simulink model "Simulation"  (R2014a)
settings: Solver=ode3  SolverMode=SingleTasking  StartTime=0.0  StopTime=5000.0  RelTol=1e-3
settings Model: ExtModeTrigDuration=2  Creator=beaverl  LastModifiedBy=beaverl
settings OptimizationCC: OptimizeModelRefInitCode=on  LifeSpan=1
settings DebuggingCC: UnderspecifiedInitializationDetection=Classic  SolverPrmCheckMsg=none
settings HardwareCC: ProdBitPerInt=16  ProdBitPerPointer=8  ProdIntDivRoundTo=Zero  ProdEndianess=LittleEndian  ProdWordSize=8  ProdHWDeviceType=Atmel->AVR
settings RTWCC: SystemTargetFile=realtime.tlc  GenerateMakefile=off  TemplateMakefile=realtime.tmf  Description=Run on Target Hardware  RTWVerbose=off  ProcessScript=realtime_make_rtw_hook
settings STFCustomTargetCC: TargetLibSuffix=.a  GenerateSampleERTMain=on  ConcurrentExecutionCompliant=off  GeneratePreprocessorConditionals=Use local settings  ERTCustomFileBanners=on  SupportNonInlinedSFcns=off  SupportVariableSizeSignals=on  MATLABClassNameForMDSCustomization=Simulink.SoftwareTarget.ERTCustomization  GRTInterface=off  SystemTargetFile=realtime.tlc
settings ERTTargetCC: CombineOutputUpdateFcns=off  SupportContinuousTime=on  SupportVariableSizeSignals=on  ExtModeTransport=3  ExtModeMexFile=ext_serial_win32_comm  ExtModeMexArgs=0 1 9600  ERTSrcFileBannerTemplate=realtime_code_template.cgt  ERTHdrFileBannerTemplate=realtime_code_template.cgt  ERTDataSrcFileTemplate=realtime_code_template.cgt  ERTDataHdrFileTemplate=realtime_code_template.cgt  ERTCustomFileTemplate=realtime_file_process.tlc

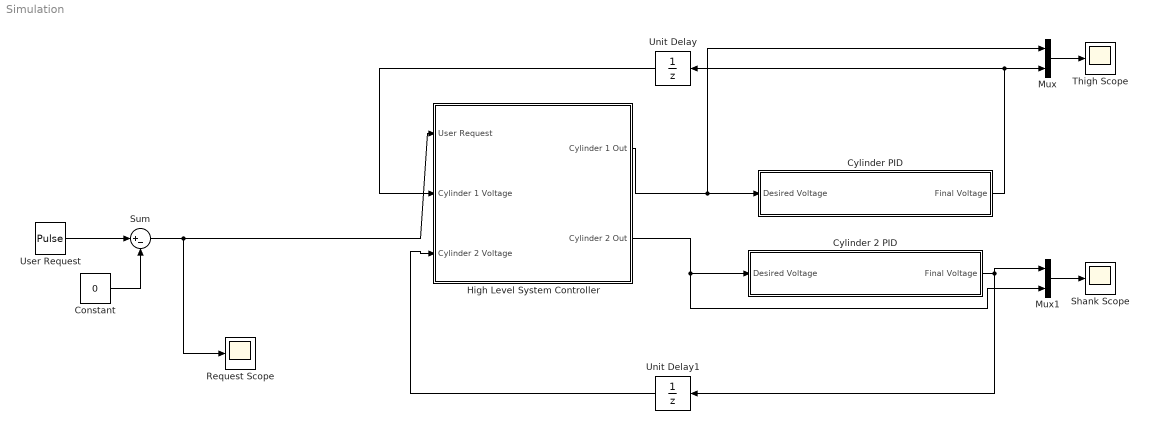
== system Simulation ==
  Constant : Constant  Value=0
  Cylinder 2 PID : Subsystem
  Cylinder PID : Subsystem
  High Level System Controller : Subsystem
  Mux : Mux  Inputs=2
  Mux1 : Mux  Inputs=2
  Request Scope : Scope
      settings: TimeRange=1  YMin=0.95  YMax=1.05
  Shank Scope : Scope
      settings: TimeRange=1  YMin=1.88  YMax=2  SaveName=ScopeData6
  Sum : Sum  Inputs=|+-
  Thigh Scope : Scope
      settings: TimeRange=1  YMin=1.88  YMax=2
  Unit Delay : UnitDelay  SampleTime=-1
  Unit Delay1 : UnitDelay  SampleTime=-1
  User Request : DiscretePulseGenerator  PulseType=Time based  Period=250  PulseWidth=50
  wires:
  High Level System Controller/1(Cylinder 1 Out) -> Mux/1, Cylinder PID/1(Desired Voltage)
  Mux/1 -> Thigh Scope/1
  Unit Delay/1 -> High Level System Controller/2(Cylinder 1 Voltage)
  User Request/1 -> Sum/1
  Constant/1 -> Sum/2
  Sum/1 -> Request Scope/1, High Level System Controller/1(User Request)
  Cylinder PID/1(Final Voltage) -> Unit Delay/1, Mux/2
  High Level System Controller/2(Cylinder 2 Out) -> Mux1/2, Cylinder 2 PID/1(Desired Voltage)
  Cylinder 2 PID/1(Final Voltage) -> Unit Delay1/1, Mux1/1
  Unit Delay1/1 -> High Level System Controller/3(Cylinder 2 Voltage)
  Mux1/1 -> Shank Scope/1

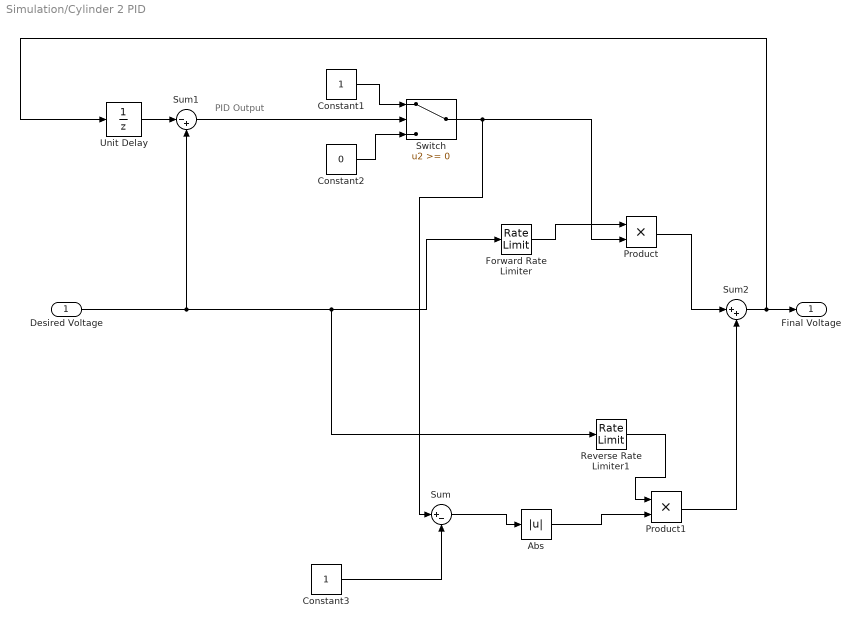
== system Simulation/Cylinder 2 PID ==
  note: PID Output
  Desired Voltage : Inport
  Abs : Abs
  Constant1 : Constant
  Constant2 : Constant  Value=0
  Constant3 : Constant
  Forward Rate Limiter : RateLimiter  RisingSlewLimit=0.0015  FallingSlewLimit=-0.0015  SampleTimeMode=inherited
  Product : Product
  Product1 : Product
  Reverse Rate Limiter1 : RateLimiter  RisingSlewLimit=0.015  FallingSlewLimit=-0.015  SampleTimeMode=inherited
  Sum : Sum  Inputs=|+-
  Sum1 : Sum  Inputs=|-+
  Sum2 : Sum  Inputs=|++
  Switch : Switch
  Unit Delay : UnitDelay  SampleTime=-1
  Final Voltage : Outport
  wires:
  Desired Voltage/1 -> Sum1/2, Reverse Rate Limiter1/1, Forward Rate Limiter/1
  Reverse Rate Limiter1/1 -> Product1/1
  Forward Rate Limiter/1 -> Product/1
  Unit Delay/1 -> Sum1/1
  Sum1/1 -> Switch/2
  Constant1/1 -> Switch/1
  Constant2/1 -> Switch/3
  Switch/1 -> Sum/1, Product/2
  Product/1 -> Sum2/1
  Sum2/1 -> Unit Delay/1, Final Voltage/1
  Sum/1 -> Abs/1
  Abs/1 -> Product1/2
  Constant3/1 -> Sum/2
  Product1/1 -> Sum2/2

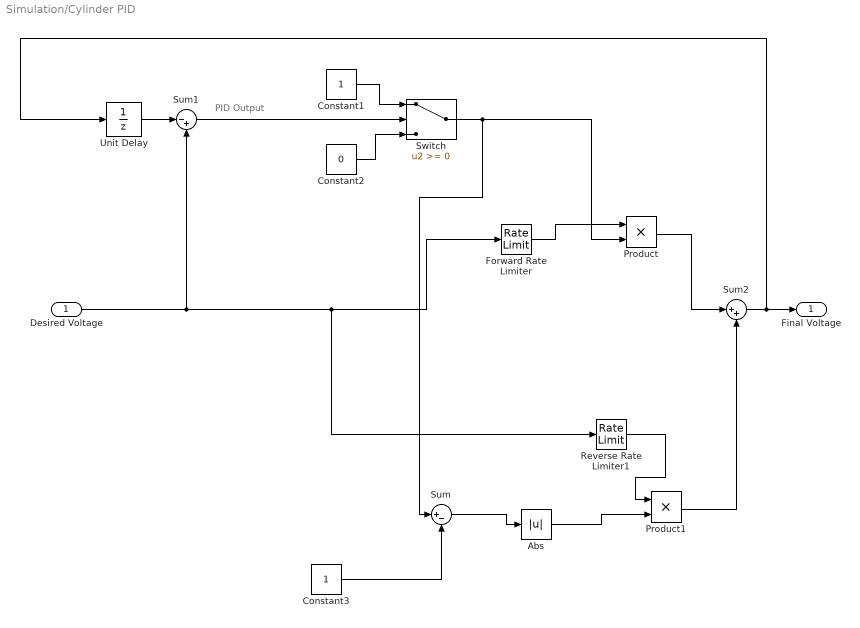
== system Simulation/Cylinder PID ==
  note: PID Output
  Desired Voltage : Inport
  Abs : Abs
  Constant1 : Constant
  Constant2 : Constant  Value=0
  Constant3 : Constant
  Forward Rate Limiter : RateLimiter  RisingSlewLimit=0.0015  FallingSlewLimit=-0.0015  SampleTimeMode=inherited
  Product : Product
  Product1 : Product
  Reverse Rate Limiter1 : RateLimiter  RisingSlewLimit=0.05  FallingSlewLimit=-0.05  SampleTimeMode=inherited
  Sum : Sum  Inputs=|+-
  Sum1 : Sum  Inputs=|-+
  Sum2 : Sum  Inputs=|++
  Switch : Switch
  Unit Delay : UnitDelay  SampleTime=-1
  Final Voltage : Outport
  wires:
  Desired Voltage/1 -> Sum1/2, Reverse Rate Limiter1/1, Forward Rate Limiter/1
  Reverse Rate Limiter1/1 -> Product1/1
  Forward Rate Limiter/1 -> Product/1
  Unit Delay/1 -> Sum1/1
  Sum1/1 -> Switch/2
  Constant1/1 -> Switch/1
  Constant2/1 -> Switch/3
  Switch/1 -> Sum/1, Product/2
  Product/1 -> Sum2/1
  Sum2/1 -> Unit Delay/1, Final Voltage/1
  Sum/1 -> Abs/1
  Abs/1 -> Product1/2
  Constant3/1 -> Sum/2
  Product1/1 -> Sum2/2

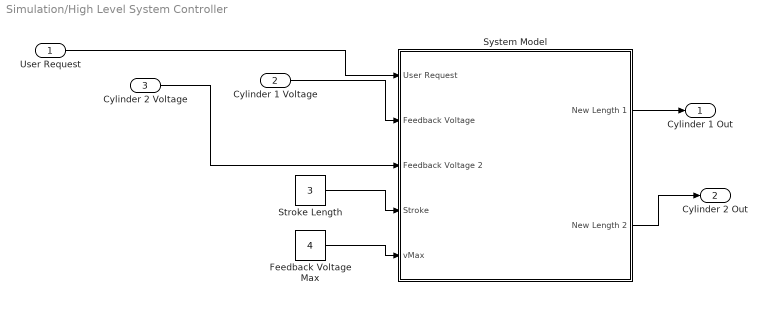
== system Simulation/High Level System Controller ==
  User Request : Inport
  Cylinder 1 Voltage : Inport  Port=2  OutDataTypeStr=double
  Cylinder 2 Voltage : Inport  Port=3  OutDataTypeStr=double
  Feedback Voltage Max : Constant  Value=4
  Stroke Length : Constant  Value=3
  System Model : Subsystem
  Cylinder 1 Out : Outport
  Cylinder 2 Out : Outport  Port=2
  wires:
  Cylinder 1 Voltage/1 -> System Model/2(Feedback Voltage)
  Stroke Length/1 -> System Model/4(Stroke)
  Feedback Voltage Max/1 -> System Model/5(vMax)
  User Request/1 -> System Model/1(User Request)
  System Model/1(New Length 1) -> Cylinder 1 Out/1
  System Model/2(New Length 2) -> Cylinder 2 Out/1
  Cylinder 2 Voltage/1 -> System Model/3(Feedback Voltage 2)

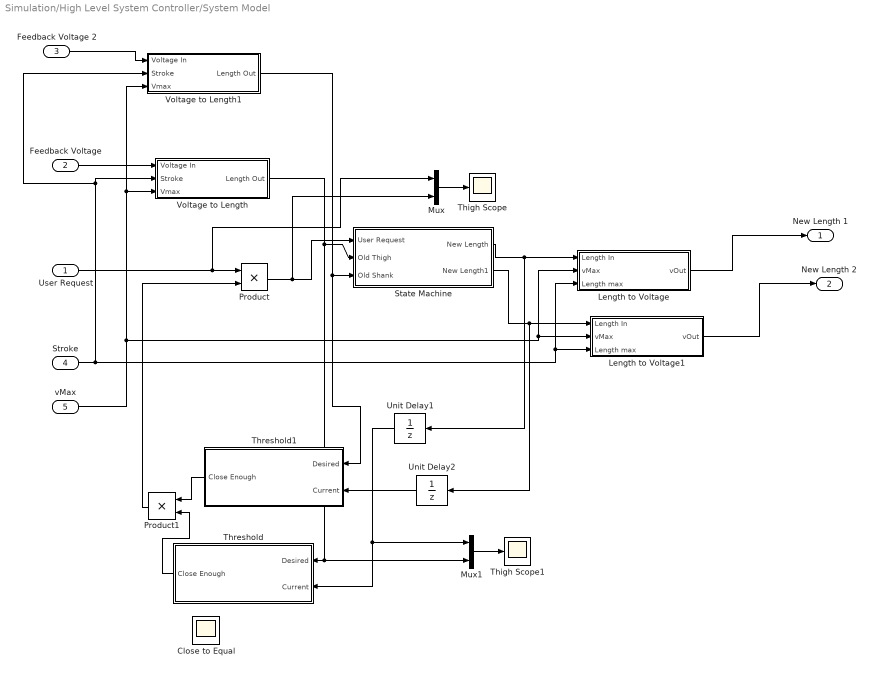
== system Simulation/High Level System Controller/System Model ==
  User Request : Inport
  Feedback Voltage : Inport  Port=2
  Feedback Voltage 2 : Inport  Port=3
  Stroke : Inport  Port=4
  vMax : Inport  Port=5
  Close to Equal : Scope
      settings: TimeRange=1  YMin=2.53334  YMax=2.8  SaveName=ScopeData5
  Length to Voltage : Subsystem
  Length to Voltage1 : Subsystem
  Mux : Mux  Inputs=2
  Mux1 : Mux  Inputs=2
  Product : Product
  Product1 : Product
  State Machine : Subsystem
  Thigh Scope : Scope
      settings: TimeRange=1  YMin=2.53334  YMax=2.8  SaveName=ScopeData3
  Thigh Scope1 : Scope
      settings: TimeRange=1  YMin=2.53334  YMax=2.8  SaveName=ScopeData4
  Threshold : Subsystem
  Threshold1 : Subsystem
  Unit Delay1 : UnitDelay  SampleTime=-1
  Unit Delay2 : UnitDelay  SampleTime=-1
  Voltage to Length : Subsystem
  Voltage to Length1 : Subsystem
  New Length 1 : Outport  OutDataTypeStr=double
  New Length 2 : Outport  Port=2  OutDataTypeStr=double
  wires:
  Feedback Voltage/1 -> Voltage to Length/1(Voltage In)
  Length to Voltage/1(vOut) -> New Length 1/1
  Stroke/1 -> Length to Voltage1/3(Length max), Length to Voltage/3(Length max), Voltage to Length1/2(Stroke), Voltage to Length/2(Stroke)
  vMax/1 -> Voltage to Length1/3(Vmax), Voltage to Length/3(Vmax), Length to Voltage/2(vMax), Length to Voltage1/2(vMax)
  State Machine/1(New Length) -> Unit Delay1/1, Length to Voltage/1(Length In)
  Voltage to Length/1(Length Out) -> Mux1/2, Threshold/1(Desired), State Machine/2(Old Thigh)
  Product/1 -> Mux/2, State Machine/1(User Request)
  User Request/1 -> Mux/1, Product/1
  Unit Delay1/1 -> Threshold/2(Current), Mux1/1
  Mux/1 -> Thigh Scope/1
  Mux1/1 -> Thigh Scope1/1
  Length to Voltage1/1(vOut) -> New Length 2/1
  State Machine/2(New Length1) -> Unit Delay2/1, Length to Voltage1/1(Length In)
  Feedback Voltage 2/1 -> Voltage to Length1/1(Voltage In)
  Voltage to Length1/1(Length Out) -> Threshold1/1(Desired), State Machine/3(Old Shank)
  Unit Delay2/1 -> Threshold1/2(Current)
  Threshold/1(Close Enough) -> Product1/2
  Threshold1/1(Close Enough) -> Product1/1
  Product1/1 -> Product/2

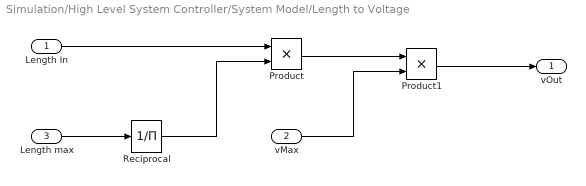
== system Simulation/High Level System Controller/System Model/Length to Voltage ==
  Length In : Inport
  vMax : Inport  Port=2
  Length max : Inport  Port=3
  Product : Product  OutDataTypeStr=Inherit: Same as first input
  Product1 : Product  OutDataTypeStr=Inherit: Same as first input
  Reciprocal : Product  Inputs=/  SaturateOnIntegerOverflow=on  RndMeth=Zero
  vOut : Outport
  wires:
  Length In/1 -> Product/1
  Reciprocal/1 -> Product/2
  Length max/1 -> Reciprocal/1
  Product/1 -> Product1/1
  vMax/1 -> Product1/2
  Product1/1 -> vOut/1

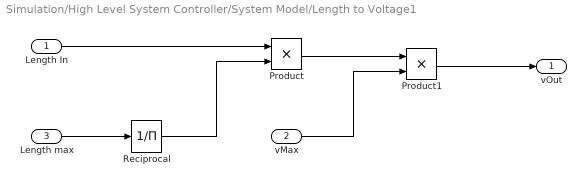
== system Simulation/High Level System Controller/System Model/Length to Voltage1 ==
  Length In : Inport
  vMax : Inport  Port=2
  Length max : Inport  Port=3
  Product : Product  OutDataTypeStr=Inherit: Same as first input
  Product1 : Product  OutDataTypeStr=Inherit: Same as first input
  Reciprocal : Product  Inputs=/  SaturateOnIntegerOverflow=on  RndMeth=Zero
  vOut : Outport
  wires:
  Length In/1 -> Product/1
  Reciprocal/1 -> Product/2
  Length max/1 -> Reciprocal/1
  Product/1 -> Product1/1
  vMax/1 -> Product1/2
  Product1/1 -> vOut/1

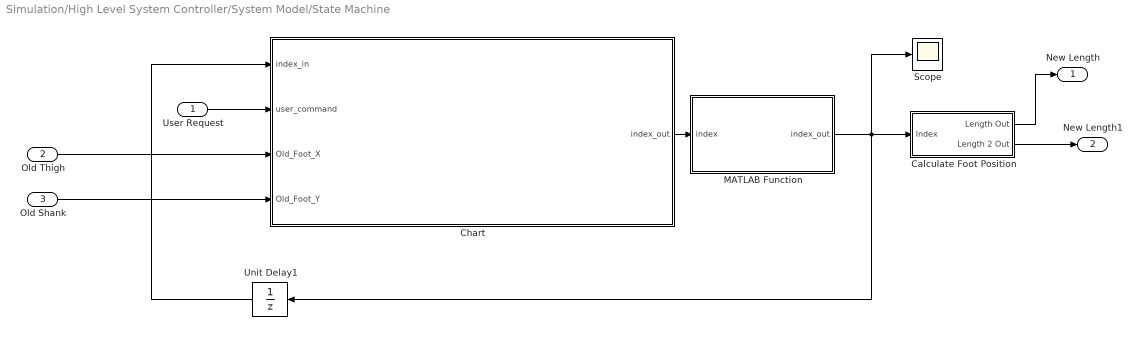
== system Simulation/High Level System Controller/System Model/State Machine ==
  User Request : Inport
  Old Thigh : Inport  Port=2
  Old Shank : Inport  Port=3
  Calculate Foot Position : Subsystem
  Chart : Stateflow chart  TreatAsAtomicUnit=on
  MATLAB Function : MATLAB Function  TreatAsAtomicUnit=on
  Scope : Scope
      settings: SaveName=ScopeData2
  Unit Delay1 : UnitDelay  SampleTime=-1
  New Length : Outport
  New Length1 : Outport  Port=2
  wires:
  User Request/1 -> Chart/2(user_command)
  Calculate Foot Position/1(Length Out) -> New Length/1
  Old Thigh/1 -> Chart/3(Old_Foot_X)
  Unit Delay1/1 -> Chart/1(index_in)
  Chart/1(index_out) -> MATLAB Function/1(index)
  MATLAB Function/1(index_out) -> Unit Delay1/1, Scope/1, Calculate Foot Position/1(Index)
  Old Shank/1 -> Chart/4(Old_Foot_Y)
  Calculate Foot Position/2(Length 2 Out) -> New Length1/1

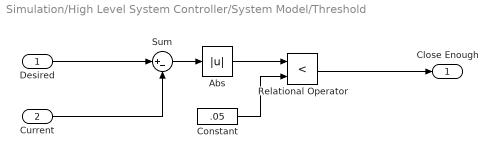
== system Simulation/High Level System Controller/System Model/Threshold ==
  Desired : Inport
  Current : Inport  Port=2
  Abs : Abs
  Constant : Constant  Value=.05
  Relational Operator : RelationalOperator  Operator=<  OutDataTypeStr=boolean
  Sum : Sum  Inputs=|+-
  Close Enough : Outport
  wires:
  Desired/1 -> Sum/1
  Current/1 -> Sum/2
  Sum/1 -> Abs/1
  Constant/1 -> Relational Operator/2
  Relational Operator/1 -> Close Enough/1
  Abs/1 -> Relational Operator/1

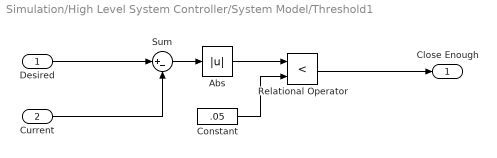
== system Simulation/High Level System Controller/System Model/Threshold1 ==
  Desired : Inport
  Current : Inport  Port=2
  Abs : Abs
  Constant : Constant  Value=.05
  Relational Operator : RelationalOperator  Operator=<  OutDataTypeStr=boolean
  Sum : Sum  Inputs=|+-
  Close Enough : Outport
  wires:
  Desired/1 -> Sum/1
  Current/1 -> Sum/2
  Sum/1 -> Abs/1
  Constant/1 -> Relational Operator/2
  Relational Operator/1 -> Close Enough/1
  Abs/1 -> Relational Operator/1

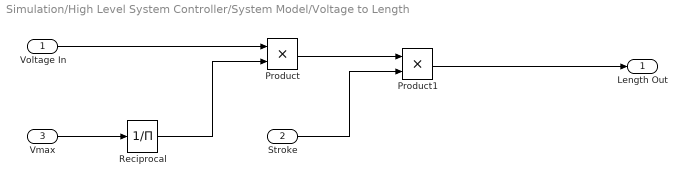
== system Simulation/High Level System Controller/System Model/Voltage to Length ==
  Voltage In : Inport
  Stroke : Inport  Port=2
  Vmax : Inport  Port=3
  Product : Product
  Product1 : Product
  Reciprocal : Product  Inputs=/  SaturateOnIntegerOverflow=on  RndMeth=Zero
  Length Out : Outport
  wires:
  Voltage In/1 -> Product/1
  Reciprocal/1 -> Product/2
  Vmax/1 -> Reciprocal/1
  Product/1 -> Product1/1
  Stroke/1 -> Product1/2
  Product1/1 -> Length Out/1

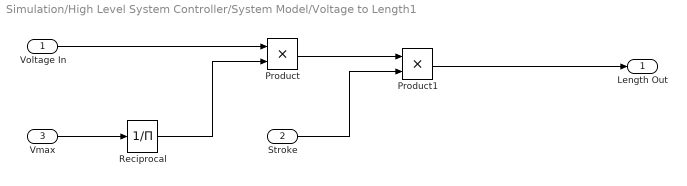
== system Simulation/High Level System Controller/System Model/Voltage to Length1 ==
  Voltage In : Inport
  Stroke : Inport  Port=2
  Vmax : Inport  Port=3
  Product : Product
  Product1 : Product
  Reciprocal : Product  Inputs=/  SaturateOnIntegerOverflow=on  RndMeth=Zero
  Length Out : Outport
  wires:
  Voltage In/1 -> Product/1
  Reciprocal/1 -> Product/2
  Vmax/1 -> Reciprocal/1
  Product/1 -> Product1/1
  Stroke/1 -> Product1/2
  Product1/1 -> Length Out/1

== system Simulation/High Level System Controller/System Model/State Machine/Calculate Foot Position ==
  Index : Inport
  MATLAB Function : MATLAB Function  TreatAsAtomicUnit=on
  Length Out : Outport
  Length 2 Out : Outport  Port=2
  wires:
  MATLAB Function/1(x1) -> Length Out/1
  Index/1 -> MATLAB Function/1(index)
  MATLAB Function/2(x2) -> Length 2 Out/1

== matlab function Simulation/High Level System Controller/System Model/State Machine/Calculate Foot Position/MATLAB Function ==
  data: x1 output; index input; x2 output
function [x1, x2]  = LookupTable(index)
%#codegen
indexTemp = index;
if(index < 1)
    indexTemp = 1;
elseif(index > 10)
    indexTemp = 10;
end;
Array = [1:0.25:2, 2:-0.25:1];

x1 = Array(indexTemp);
x2 = 2 - x1;

== stateflow chart Simulation/High Level System Controller/System Model/State Machine/Chart ==
  state Idle
    entry: index_out = index_in;
  state Reverse
    entry: index_out = index_in - 1;
    during: index_out = index_in-1;
  state Forward
    entry: index_out = index_in + 1;
    during: index_out = index_in + 1;
  Reverse -> Idle : [user_command ~= -1]
  (default) -> Idle
  Idle -> Forward [order 1] : [user_command == 1]
  Forward -> Idle : [user_command ~= 1]
  Idle -> Reverse [order 2] : [user_command == -1]
  data: index_in input; user_command input; index_out output; Old_Foot_X input; Old_Foot_Y input

== matlab function Simulation/High Level System Controller/System Model/State Machine/MATLAB Function ==
  data: index_out output; index input
function index_out = ClampIndex(index)
%#codegen
index_out = index;
if index > 10
    index_out = 1;
end
if index < 1
    index_out = 10;
end
